simulink model "Task_1"  (R2021b)
settings: Solver=ode23tb  StartTime=0.0  StopTime=5000  RelTol=1e-3
undefined symbols (not defined in the file): Ion, Lithium
libraries: eeStairGenerator x3, spsBatteryLib x2, spsControlledCurrentSourceLib x2, spspowerguiLib x1
settings Model: Creator=eee  LastModifiedBy=casum
settings SolverCC: AlgebraicLoopSolver=TrustRegion

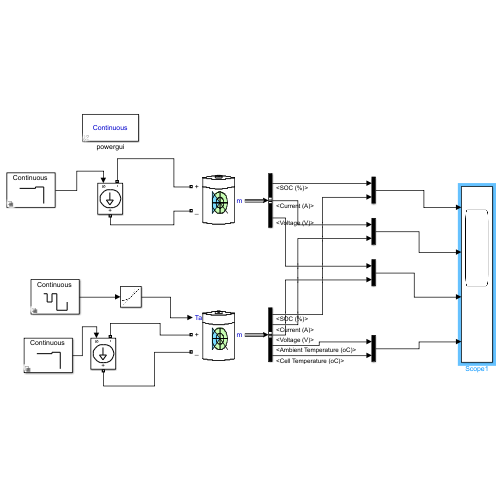
[thumbnail: Simulink's stored preview of the top-level diagram]
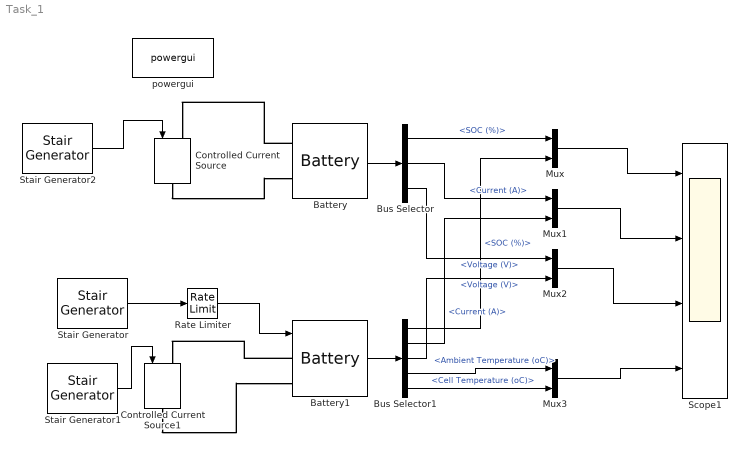
== system Task_1 ==
  Battery : spsBatteryLib/Battery  BatType=Lithium-Ion  ShowTempParam=off  ThermalPreset=no  ShowAgeParam=off  NomV=7.2  NomQ=5.4  SOC=100  Batt_Tr=30  PresetModel=on  MaxQ=5.4  MinV=5.4  FullV=8.3807  Dis_rate=2.3478  R=0.013333  Normal_OP=4.8835  expZone="[7.7788      0.2653]"  current=[6.5 13 32.5]  Units=Time  Tci=20  NomT=20  T2=-30  MaxQ2=4.8  FullV2=7.1  Normal_OP2=5.655  expZone2="[6.58           1]"  Rca=0.6  ti=2000  Dp=0  Neq0=0  Tsim=1e6  Ta1=25  Qeol=5.4*0.9  Reol=0.013333*1.2  Char_age=[2.3478, 3]  Dis_age=[2.3478, 10]  N1=1500  N2=10500  N3=1000  N4=1400  Ta2=45  N5=950
  Battery1 : spsBatteryLib/Battery  BatType=Lithium-Ion  ShowTempParam=on  ThermalPreset="12.8V  40Ah  (LiFeMgPO4)"  ShowAgeParam=off  NomV=12.6  NomQ=40  SOC=100  Batt_Tr=30  PresetModel=off  MaxQ=40  MinV=10.5  FullV=13.8  Dis_rate=20  R=0.015  Normal_OP=30.14  expZone="[13.1          0.5]"  current=[6.5 13 32.5]  Units=Time  Tci=20  NomT=20  T2=0  MaxQ2=36  FullV2=13  Normal_OP2=11.7  expZone2="[12.67            4]"  Rca=0.6411  ti=4880  Dp=0  Neq0=0  Tsim=1e6  Ta1=25  Qeol=5.4*0.9  Reol=0.013333*1.2  Char_age=[2.3478, 3]  Dis_age=[2.3478, 10]  N1=1500  N2=10500  N3=1000  N4=1400  Ta2=45  N5=950
  Bus Selector : BusSelector  OutputSignals=SOC (%),Current (A),Voltage (V)
  Bus Selector1 : BusSelector  OutputSignals=SOC (%),Current (A),Voltage (V),Ambient Temperature (oC),Cell Temperature (oC)
  Controlled Current Source : spsControlledCurrentSourceLib/Controlled Current Source  Initialize=on  Source_Type=AC  Amplitude=0  Phase=0  Frequency=0  Measurements=None
  Controlled Current Source1 : spsControlledCurrentSourceLib/Controlled Current Source  Initialize=on  Source_Type=AC  Amplitude=0  Phase=0  Frequency=0  Measurements=None
  Mux{,1..3} (4 alike) : Mux  Inputs=2
  Rate Limiter : RateLimiter  RisingSlewLimit=0.5  FallingSlewLimit=-0.5  SampleTimeMode=inherited
  Scope1 : Scope  NumInputPorts=4
  Stair Generator : eeStairGenerator/Stair Generator  LabelModeActiveChoice=Continuous  TimeInput=[0 500 1250 2000 3500]  AmplitudeInput=[20 0 20 -20 0]  SampleTime=0  RepeatPattern=off  OutDataTypeStr=double
      settings: SourceProductBaseCode=PS
  Stair Generator1 : eeStairGenerator/Stair Generator  LabelModeActiveChoice=Continuous  TimeInput=[0 2000 3000]  AmplitudeInput=[15 20 -35]  SampleTime=0  RepeatPattern=off  OutDataTypeStr=double
      settings: SourceProductBaseCode=PS
  Stair Generator2 : eeStairGenerator/Stair Generator  LabelModeActiveChoice=Continuous  TimeInput=[0 2000 3000]  AmplitudeInput=[15 20 -35]  SampleTime=0  RepeatPattern=off  OutDataTypeStr=double
      settings: SourceProductBaseCode=PS
  powergui : spspowerguiLib/powergui  Priority=1  SimulationMode=Continuous  SampleTime=50e-6  frequency=60  Iterations=50  frequencyindice=0  Pbase=100e6  ErrMax=1e-4  UnitsV=kV  UnitsW=MW  buscounter=0  FunctionMessages=off  echomessages=off  EnableUseOfTLC=off  CurrentSourceSwitches=off  DisableSnubberDevices=off  DisableRonSwitches=off  DisableVfSwitches=off  DisplayEquations=off  AutomaticDiscreteSolvers=off  SolverType=Tustin/Backward Euler (TBE)  Interpol=off  ExternalGateDelay=off  methode=off  Ts=100  x0status=blocks  SPID=on  SwTol=0  HookPort=off  NonlinearTolerance=1e-4  nMaxIteration=100  ContinueOnMaxIteration=off  RestoreLinks=warning  ResistiveCurrentMeasurement=off  Frange=[0:2:500]  Ylog=off  Xlog=on  ShowGrid=off  save=off  variable=ZData  structure=0  ZoomFFT=off  StartTime=0.0  cycles=1  DisplayStyle=1  fundamental=60  FreqAxis=off  MaxFrequency=1000  frequencyindicesteady=1  RmsSteady=1  display=off
  wires:
  Battery/1 -> Bus Selector/1
  Battery1/1 -> Bus Selector1/1
  Stair Generator/1 -> Rate Limiter/1
  Rate Limiter/1 -> Battery1/1
  Bus Selector/1 -> Mux/1  "<SOC (%)>"
  Bus Selector1/1 -> Mux/2  "<SOC (%)>"
  Bus Selector/2 -> Mux1/1  "<Current (A)>"
  Bus Selector1/2 -> Mux1/2  "<Current (A)>"
  Bus Selector/3 -> Mux2/1  "<Voltage (V)>"
  Bus Selector1/3 -> Mux2/2  "<Voltage (V)>"
  Bus Selector1/4 -> Mux3/1  "<Ambient Temperature (oC)>"
  Bus Selector1/5 -> Mux3/2  "<Cell Temperature (oC)>"
  Mux/1 -> Scope1/1
  Mux1/1 -> Scope1/2
  Mux2/1 -> Scope1/3
  Mux3/1 -> Scope1/4
  Stair Generator1/1 -> Controlled Current Source1/1
  Stair Generator2/1 -> Controlled Current Source/1
  connections:
  Battery/LConn1 -- Controlled Current Source/LConn1
  Controlled Current Source/RConn1 -- Battery/LConn2
  Battery1/LConn1 -- Controlled Current Source1/LConn1
  Controlled Current Source1/RConn1 -- Battery1/LConn2
